simulink model "projekat"  (R2021a)
settings: Solver=FixedStepAuto  StartTime=0.0  StopTime=4000  FixedStep=0.1  RelTol=1e-3
libraries: fuzblock x4
settings Model: Creator=anazo  LastModifiedBy=anazo

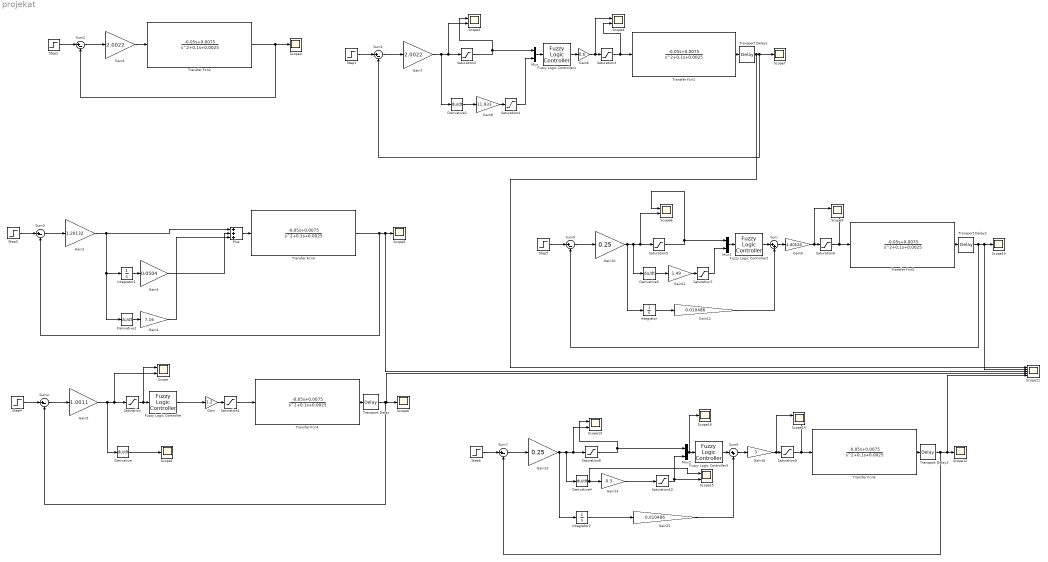
== system projekat ==
  Derivative{,1..4} (5 alike) : Derivative
  Fuzzy Logic Controller : fuzblock/Fuzzy Logic  Controller  FIS='greska0.fis'  OutputSampleNumber=101  DataType=double  FuzzifiedInputs=off  RuleFiringStrengths=off  RuleOutputs=off  AggregatedOutputs=off  SimulateUsing=Interpreted execution  OutOfRangeInputValueMessage=warning  NoRuleFiredMessage=warning  EmptyOutputFuzzySetMessage=warning
  Fuzzy Logic Controller1 : fuzblock/Fuzzy Logic  Controller  FIS='greska.fis'  OutputSampleNumber=101  DataType=double  FuzzifiedInputs=off  RuleFiringStrengths=off  RuleOutputs=off  AggregatedOutputs=off  SimulateUsing=Interpreted execution  OutOfRangeInputValueMessage=warning  NoRuleFiredMessage=warning  EmptyOutputFuzzySetMessage=warning
  Fuzzy Logic Controller2 : fuzblock/Fuzzy Logic  Controller  FIS='greska.fis'  OutputSampleNumber=101  DataType=double  FuzzifiedInputs=off  RuleFiringStrengths=off  RuleOutputs=off  AggregatedOutputs=off  SimulateUsing=Interpreted execution  OutOfRangeInputValueMessage=warning  NoRuleFiredMessage=warning  EmptyOutputFuzzySetMessage=warning
  Fuzzy Logic Controller3 : fuzblock/Fuzzy Logic  Controller  FIS='greskanln.fis'  OutputSampleNumber=101  DataType=double  FuzzifiedInputs=off  RuleFiringStrengths=off  RuleOutputs=off  AggregatedOutputs=off  SimulateUsing=Interpreted execution  OutOfRangeInputValueMessage=warning  NoRuleFiredMessage=warning  EmptyOutputFuzzySetMessage=warning
  Gain : Gain  Gain=1.2
  Gain1 : Gain  Gain=2.0022
  Gain10 : Gain  Gain=0.25
  Gain11 : Gain  Gain=1.49
  Gain12 : Gain  Gain=0.010486
  Gain13 : Gain  Gain=0.25
  Gain14 : Gain  Gain=0.3
  Gain15 : Gain  Gain=0.010486
  Gain16 : Gain  Gain=3
  Gain2 : Gain  Gain=1.20132
  Gain3 : Gain  Gain=0.0504
  Gain4 : Gain  Gain=7.16
  Gain5 : Gain  Gain=1.0011
  Gain6 : Gain  Gain=0.6
  Gain7 : Gain  Gain=2.0022
  Gain8 : Gain  Gain=11.933
  Gain9 : Gain  Gain=4.80528
  Integrator : Integrator
  Integrator1 : Integrator
  Integrator2 : Integrator
  Mux : Mux  Inputs=2
  Mux1 : Mux  Inputs=2
  Mux2 : Mux  Inputs=2
  Plus : Sum  Inputs=+++
  Saturation{,2,4..5,7..8,10} (7 alike) : Saturate  UpperLimit=1  LowerLimit=-1
  Saturation{1,3,6,9} (4 alike) : Saturate  UpperLimit=1.2  LowerLimit=-1.2
  Scope{,2,4,8..9,13..15} (8 alike) : Scope  NumInputPorts=2
  Scope{1,3,5..7,10,12,16} (8 alike) : Scope
  Scope11 : Scope  NumInputPorts=5
  Step{1,3..6} (5 alike) : Step  Time=2000  Before=-2  After=2  SampleTime=0
  Step2 : Step  Time=4000  Before=-2  After=2  SampleTime=0
  Sum : Sum  Inputs=|++
  Sum{1..5,7} (6 alike) : Sum  Inputs=|+-
  Sum6 : Sum  Inputs=|++
  Transfer Fcn{1..6} (6 alike) : TransferFcn  Numerator=[-0.05 0.0075]  Denominator=[1 0.1 0.0025]
  Transport Delay{,1..3} (4 alike) : TransportDelay  DelayTime=3.6
  wires:
  Transport Delay/1 -> Sum4/2, Scope11/4, Scope6/1
  Step4/1 -> Sum4/1
  Sum4/1 -> Gain5/1
  Derivative1/1 -> Gain4/1
  Gain4/1 -> Plus/3
  Gain3/1 -> Plus/2
  Gain2/1 -> Derivative1/1, Integrator1/1, Plus/1
  Transfer Fcn3/1 -> Sum3/2, Scope11/3, Scope5/1
  Step3/1 -> Sum3/1
  Sum3/1 -> Gain2/1
  Sum2/1 -> Gain1/1
  Transfer Fcn2/1 -> Sum2/2, Scope3/1
  Gain1/1 -> Transfer Fcn2/1
  Plus/1 -> Transfer Fcn3/1
  Integrator1/1 -> Gain3/1
  Step2/1 -> Sum2/1
  Fuzzy Logic Controller/1 -> Gain/1
  Saturation/1 -> Scope/1, Fuzzy Logic Controller/1
  Derivative/1 -> Scope1/1
  Saturation1/1 -> Transfer Fcn4/1
  Gain/1 -> Saturation1/1
  Gain5/1 -> Scope/2, Saturation/1, Derivative/1
  Transfer Fcn4/1 -> Transport Delay/1
  Sum1/1 -> Gain7/1
  Step1/1 -> Sum1/1
  Saturation3/1 -> Scope4/2, Transfer Fcn1/1
  Fuzzy Logic Controller1/1 -> Gain6/1
  Gain7/1 -> Scope2/2, Saturation2/1, Derivative2/1
  Saturation2/1 -> Mux/1, Scope2/1
  Gain6/1 -> Scope4/1, Saturation3/1
  Transfer Fcn1/1 -> Transport Delay1/1
  Mux/1 -> Fuzzy Logic Controller1/1
  Derivative2/1 -> Gain8/1
  Gain8/1 -> Saturation4/1
  Saturation4/1 -> Mux/2
  Saturation7/1 -> Mux1/2
  Mux1/1 -> Fuzzy Logic Controller2/1
  Saturation5/1 -> Mux1/1, Scope8/1
  Gain10/1 -> Integrator/1, Scope8/2, Saturation5/1, Derivative3/1
  Transfer Fcn5/1 -> Transport Delay2/1
  Saturation6/1 -> Scope9/2, Transfer Fcn5/1
  Sum5/1 -> Gain10/1
  Step5/1 -> Sum5/1
  Transport Delay2/1 -> Sum5/2, Scope11/2, Scope10/1
  Gain11/1 -> Saturation7/1
  Derivative3/1 -> Gain11/1
  Integrator/1 -> Gain12/1
  Gain9/1 -> Scope9/1, Saturation6/1
  Fuzzy Logic Controller2/1 -> Sum/1
  Sum/1 -> Gain9/1
  Gain12/1 -> Sum/2
  Transport Delay1/1 -> Scope7/1, Sum1/2, Scope11/1
  Gain15/1 -> Sum6/2
  Transport Delay3/1 -> Sum7/2, Scope11/5, Scope12/1
  Saturation10/1 -> Scope15/2, Mux2/2
  Sum6/1 -> Gain16/1
  Gain16/1 -> Scope14/1, Saturation9/1
  Saturation9/1 -> Scope14/2, Transfer Fcn6/1
  Transfer Fcn6/1 -> Transport Delay3/1
  Integrator2/1 -> Gain15/1
  Gain14/1 -> Saturation10/1
  Fuzzy Logic Controller3/1 -> Sum6/1
  Gain13/1 -> Integrator2/1, Scope13/2, Saturation8/1, Derivative4/1
  Step6/1 -> Sum7/1
  Saturation8/1 -> Mux2/1, Scope13/1
  Sum7/1 -> Gain13/1
  Mux2/1 -> Scope16/1, Fuzzy Logic Controller3/1
  Derivative4/1 -> Scope15/1, Gain14/1
